simulink model "SCex4_1simulink"  (R2024b)
settings: Solver=VariableStepAuto  StartTime=0.0  StopTime=10.0  RelTol=1e-3
libraries: simulink x1
settings Model: Creator=pedro  LastModifiedBy=pedro

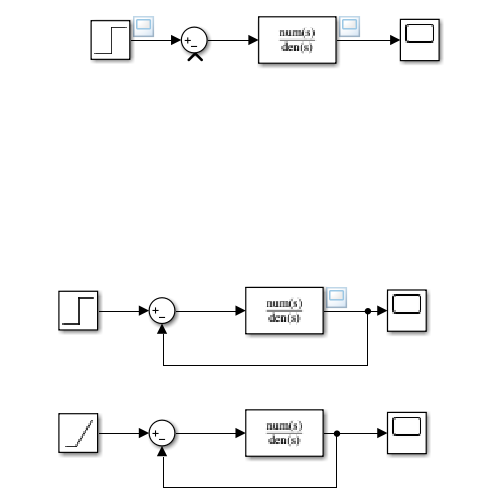
[thumbnail: Simulink's stored preview of the top-level diagram]
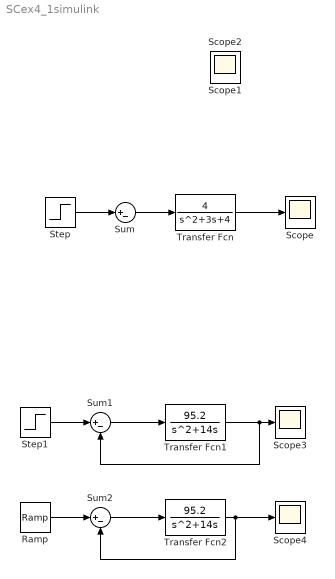
== system SCex4_1simulink ==
  Ramp : simulink/Sources/Ramp  slope=1  start=0  InitialOutput=0
  Scope{,1..4} (5 alike) : Scope
  Step : Step  SampleTime=0
  Step1 : Step  SampleTime=0
  Sum : Sum  Inputs=|+-
  Sum1 : Sum  Inputs=|+-
  Sum2 : Sum  Inputs=|+-
  Transfer Fcn : TransferFcn  Numerator=[4]  Denominator=[1 3 4]
  Transfer Fcn1 : TransferFcn  Numerator=[95.2]  Denominator=[1 14 0]
  Transfer Fcn2 : TransferFcn  Numerator=[95.2]  Denominator=[1 14 0]
  wires:
  Sum/1 -> Transfer Fcn/1
  Step/1 -> Sum/1
  Transfer Fcn/1 -> Scope/1
  Step1/1 -> Sum1/1
  Transfer Fcn1/1 -> Sum1/2, Scope3/1
  Sum1/1 -> Transfer Fcn1/1
  Sum2/1 -> Transfer Fcn2/1
  Transfer Fcn2/1 -> Sum2/2, Scope4/1
  Ramp/1 -> Sum2/1
